simulink model "specificapwm"  (R2022b)
settings: Solver=ode45  StartTime=0.0  StopTime=10.0  RelTol=1e-3
undefined symbols (not defined in the file or in its folder): pwr
libraries: simulink x5
settings Model: Creator=tborlina  LastModifiedBy=gotta

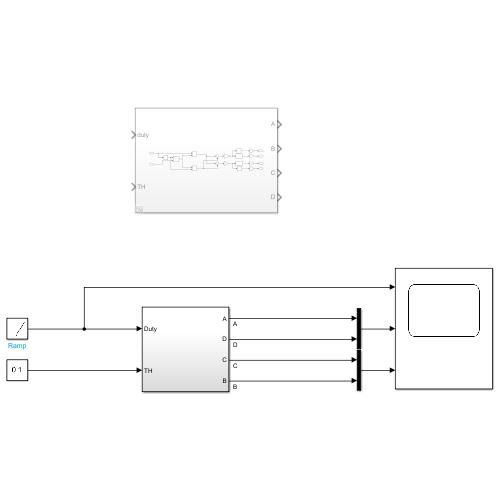
[thumbnail: Simulink's stored preview of the top-level diagram]
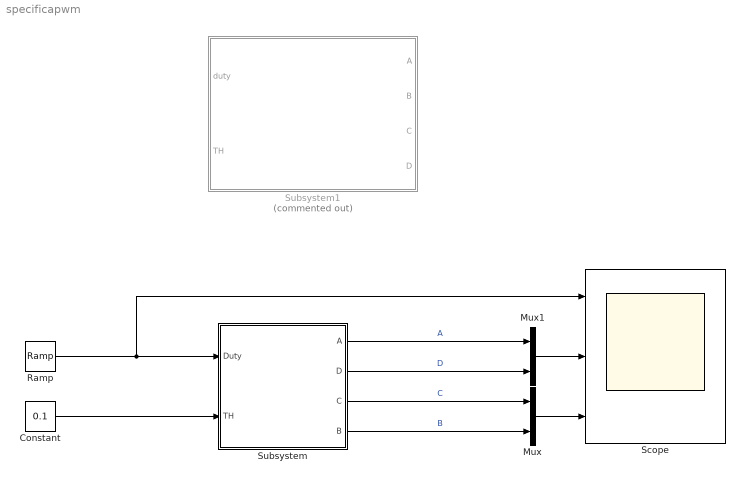
== system specificapwm ==
  Constant : Constant  Value=0.1
  Mux : Mux  Inputs=2
  Mux1 : Mux  Inputs=2
  Ramp : simulink/Sources/Ramp  slope=0.2  start=0  InitialOutput=-1
  Scope : Scope  NumInputPorts=3
  Subsystem : Subsystem
  Subsystem1 : Subsystem  Commented=on
  wires:
  Constant/1 -> Subsystem/2(TH)
  Ramp/1 -> Scope/1, Subsystem/1(Duty)
  Mux/1 -> Scope/3
  Subsystem/1(A) -> Mux1/1  "A"
  Subsystem/2(D) -> Mux1/2  "D"
  Mux1/1 -> Scope/2
  Subsystem/3(C) -> Mux/1  "C"
  Subsystem/4(B) -> Mux/2  "B"

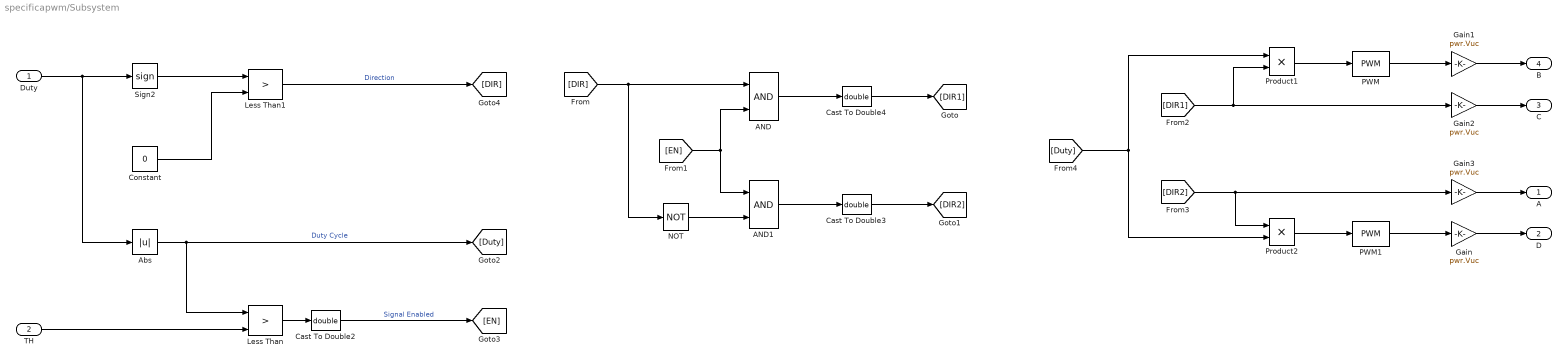
== system specificapwm/Subsystem ==
  Duty : Inport
  TH : Inport  Port=2
  AND : Logic  IconShape=distinctive  AllPortsSameDT=off  OutDataTypeStr=boolean
  AND1 : Logic  IconShape=distinctive  AllPortsSameDT=off  OutDataTypeStr=boolean
  Abs : Abs  SaturateOnIntegerOverflow=off
  Cast To Double2 : DataTypeConversion  OutDataTypeStr=double  SaturateOnIntegerOverflow=off  RndMeth=Floor
  Cast To Double3 : DataTypeConversion  OutDataTypeStr=double  SaturateOnIntegerOverflow=off  RndMeth=Floor
  Cast To Double4 : DataTypeConversion  OutDataTypeStr=double  SaturateOnIntegerOverflow=off  RndMeth=Floor
  Constant : Constant  Value=0
  Gain{,1..3} (4 alike) : Gain  Gain=pwr.Vuc
  Less Than : RelationalOperator  Operator=>  OutDataTypeStr=boolean  RndMeth=Simplest  InputSameDT=off
  Less Than1 : RelationalOperator  Operator=>  OutDataTypeStr=boolean  RndMeth=Simplest  InputSameDT=off
  NOT : Logic  Operator=NOT  IconShape=distinctive  AllPortsSameDT=off  OutDataTypeStr=boolean
  PWM : simulink/Discontinuities/PWM  DisableCoverage=on  Period=0.1  InitialDelay=0  DisallowZeroDutyCycle=off  RunAtFixedTimeIntervals=on  SampleTime=0.001
  PWM1 : simulink/Discontinuities/PWM  DisableCoverage=on  Period=0.1  InitialDelay=0  DisallowZeroDutyCycle=off  RunAtFixedTimeIntervals=on  SampleTime=0.001
  Product1 : Product
  Product2 : Product
  Sign2 : Signum
  A : Outport
  D : Outport  Port=2
  C : Outport  Port=3
  B : Outport  Port=4
  wires:
  TH/1 -> Less Than/2
  Duty/1 -> Abs/1, Sign2/1
  Less Than/1 -> Cast To Double2/1
  Sign2/1 -> Less Than1/1
  Constant/1 -> Less Than1/2
  Abs/1 -> [Duty], Less Than/1  "Duty Cycle"
  Gain/1 -> D/1
  Gain1/1 -> B/1
  Gain2/1 -> C/1
  Gain3/1 -> A/1
  AND1/1 -> Cast To Double3/1
  AND/1 -> Cast To Double4/1
  NOT/1 -> AND1/2
  Product1/1 -> PWM/1
  Product2/1 -> PWM1/1
  Cast To Double2/1 -> [EN]  "Signal Enabled"
  Less Than1/1 -> [DIR]  "Direction"
  [DIR] -> NOT/1, AND/1
  [EN] -> AND/2, AND1/1
  Cast To Double4/1 -> [DIR1]
  Cast To Double3/1 -> [DIR2]
  [DIR1] -> Product1/2, Gain2/1
  [DIR2] -> Product2/1, Gain3/1
  [Duty] -> Product1/1, Product2/2
  PWM/1 -> Gain1/1
  PWM1/1 -> Gain/1

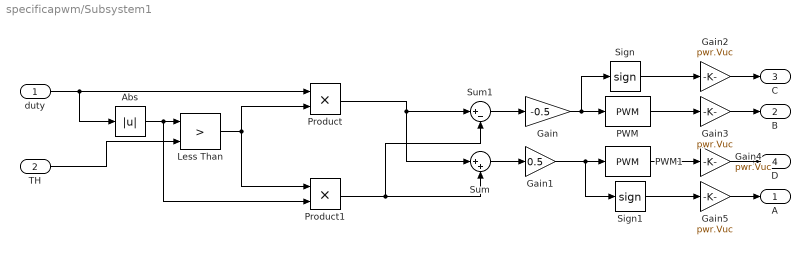
== system specificapwm/Subsystem1 ==
  duty : Inport
  TH : Inport  Port=2
  Abs : Abs  SaturateOnIntegerOverflow=off
  Gain : Gain  Gain=-0.5
  Gain1 : Gain  Gain=0.5
  Gain{2..5} (4 alike) : Gain  Gain=pwr.Vuc
  Less Than : RelationalOperator  Operator=>  OutDataTypeStr=boolean  RndMeth=Simplest  InputSameDT=off
  PWM : simulink/Discontinuities/PWM  DisableCoverage=on  Period=1  InitialDelay=0  DisallowZeroDutyCycle=off  RunAtFixedTimeIntervals=off  SampleTime=0.1
  PWM1 : simulink/Discontinuities/PWM  DisableCoverage=on  Period=1  InitialDelay=0  DisallowZeroDutyCycle=off  RunAtFixedTimeIntervals=off  SampleTime=0.1
  Product : Product
  Product1 : Product
  Sign : Signum
  Sign1 : Signum
  Sum : Sum  Inputs=|++
  Sum1 : Sum  Inputs=|+-
  A : Outport
  B : Outport  Port=2
  C : Outport  Port=3
  D : Outport  Port=4
  wires:
  Sign/1 -> Gain2/1
  Sign1/1 -> Gain5/1
  Gain1/1 -> PWM1/1, Sign1/1
  Gain/1 -> PWM/1, Sign/1
  Sum1/1 -> Gain/1
  Sum/1 -> Gain1/1
  Product1/1 -> Sum/2, Sum1/2
  Product/1 -> Sum1/1, Sum/1
  Less Than/1 -> Product1/1, Product/2
  Abs/1 -> Less Than/1, Product1/2
  duty/1 -> Product/1, Abs/1
  TH/1 -> Less Than/2
  Gain2/1 -> C/1
  Gain3/1 -> B/1
  Gain4/1 -> D/1
  Gain5/1 -> A/1
  PWM/1 -> Gain3/1
  PWM1/1 -> Gain4/1
